simulink model "simple_AD_cont"  (R2019a)
settings: Solver=ode23tb  StartTime=0.0  StopTime=0.16  RelTol=1e-5  AbsTol=0.00001  EnableMultiTasking=on
values from neighbouring files (symbols this model uses):
  C_x1 = 10e-6    (= 1e-05)    [start.m]
  DEN_cc = Ks_curr.den{1,1}    [start.m]
  f_n = 50    [start.m]
  f_sw = 8000    [start.m]
  Id_ref = 15    [start.m]
  kic = ss(0,0,0,kic,Ts_control)    [current_controller.m]    (also in start.m = 0.042)
  L_f1 = 1.6e-3    (= 0.0016)    [start.m]
  L_f2 = 0.8e-3    (= 0.0008)    [start.m]
  Lgrid = 5e-3    (= 0.005)    [start.m]
  NUM_cc = Ks_curr.num{1,1}    [start.m]
  R_f1 = 2e-3    (= 0.002)    [start.m]
  R_f2 = 1e-3    (= 0.001)    [start.m]
  R_x1 = 0.1e-3    (= 0.0001)    [start.m]
  Rgrid = 10    [start.m]
  Ts_control = 1/f_sample    (= 6.25e-05)    [start.m]
  V_dc_ref = 700    [start.m]
  V_ffwd = -1    [start.m]
  Vg_h12 = 0*Vgrid    [start.m]
  Vg_h15 = 0*Vgrid    [start.m]
  Vg_h5 = 0*Vgrid    [start.m]
  Vg_h7 = 0*Vgrid    [start.m]
  Vgrid = 127*sqrt(2)    [start.m]
undefined symbols (not defined in the file or in its folder): C_f1, T_power
libraries: powerlib x21, simulink x2, powerlib_extras x2, powerlib_meascontrol x1
settings Model: Creator=FOR_WORK  LastModifiedBy=ityur
settings SolverCC: AutoScaleAbsTol=off
settings DataIOCC: LimitDataPoints=on  SaveFormat=Array  SignalLoggingSaveFormat=ModelDataLogs  ReturnWorkspaceOutputs=off
settings OptimizationCC: LifeSpan=inf
settings DebuggingCC: UnderspecifiedInitializationDetection=Classic  MergeDetectMultiDrivingBlocksExec=none  SolverPrmCheckMsg=warning  MultiTaskDSMMsg=warning  MultiTaskCondExecSysMsg=none  UnconnectedInputMsg=none  UnconnectedOutputMsg=none  UnconnectedLineMsg=none  StateNameClashWarn=warning  SFUnexpectedBacktrackingDiag=warning  SFNoUnconditionalDefaultTransitionDiag=warning  SFExecutionAtInitializationDiag=none  ArithmeticOperatorsInVariantConditions=warning
settings HardwareCC: ProdBitPerPointer=32  ProdBitPerSizeT=32  ProdBitPerPtrDiffT=32  ProdLargestAtomicFloat=None  ProdIntDivRoundTo=Undefined  ProdEndianess=Unspecified  ProdWordSize=32  ProdHWDeviceType=32-bit Generic
settings ModelReferenceCC: PropagateSignalLabelsOutOfModel=off
settings SFSimCC: SimUseLocalCustomCode=off
settings RTWCC: RTWUseLocalCustomCode=off
settings CodeAppCC: StateflowObjectComments=on
settings GRTTargetCC: TargetLangStandard=C89/C90 (ANSI)  GeneratePreprocessorConditionals=Disable all
settings ConfigComp: CovMetricSettings=dw  CovHtmlReporting=on  CovSaveCumulativeToWorkspaceVar=on  CovSaveSingleToWorkspaceVar=on  CovExternalEMLEnable=off  CovSFcnEnable=off
settings SimscapeCC: SimscapeNormalizeSystem=off

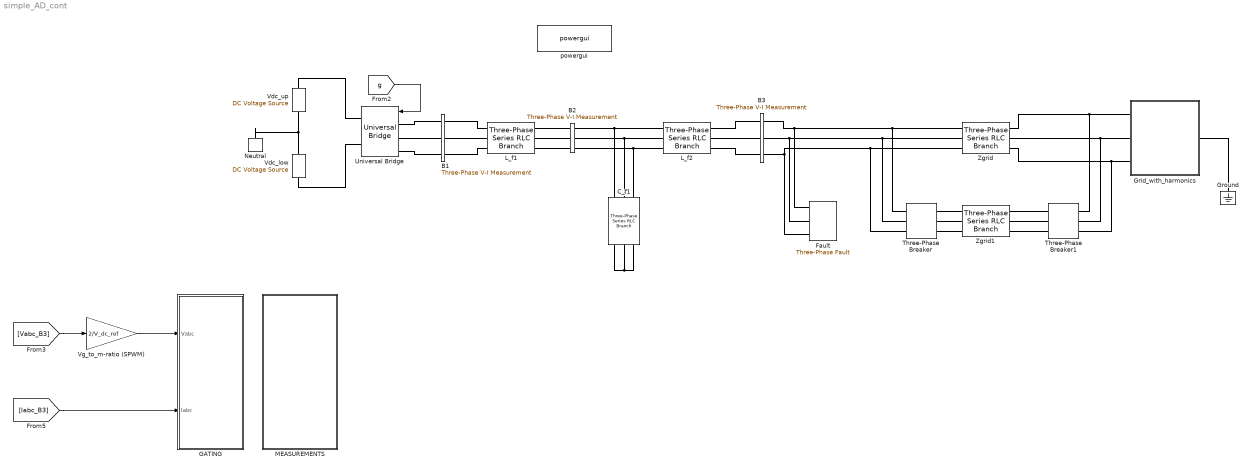
== system simple_AD_cont ==
  B1 : powerlib/Measurements/Three-Phase V-I Measurement  VoltageMeasurement=phase-to-phase  SetLabelV=on  LabelV=Vabc_B1  Vpu=off  VpuLL=off  CurrentMeasurement=yes  SetLabelI=on  LabelI=Iabc_B1  Ipu=off  Pbase=28e3  Vbase=480  OutputType=Magnitude  PhasorSimulation=off  PSBequivalent=0
      settings: SourceProductName=Simscape Electrical
  B2 : powerlib/Measurements/Three-Phase V-I Measurement  VoltageMeasurement=no  SetLabelV=on  LabelV=Vabc_B2  Vpu=off  VpuLL=off  CurrentMeasurement=yes  SetLabelI=on  LabelI=Iabc_B2  Ipu=off  Pbase=50e3  Vbase=Vi_n  OutputType=Magnitude  PhasorSimulation=off  PSBequivalent=0
      settings: SourceProductName=Simscape Electrical
  B3 : powerlib/Measurements/Three-Phase V-I Measurement  VoltageMeasurement=phase-to-ground  SetLabelV=on  LabelV=Vabc_B3  Vpu=off  VpuLL=off  CurrentMeasurement=yes  SetLabelI=on  LabelI=Iabc_B3  Ipu=off  Pbase=50e3  Vbase=Vi_n  OutputType=Magnitude  PhasorSimulation=off  PSBequivalent=0
      settings: SourceProductName=Simscape Electrical
  C_f1 : powerlib/Elements/Three-Phase Series RLC Branch  LConnTagsString=A|B|C  RConnTagsString=A|B|C  BranchType=RC  Resistance=R_x1  Inductance=L_f1  Capacitance=C_x1  Measurements=None
      settings: SourceProductName=Simscape Electrical
  Fault : powerlib/Elements/Three-Phase Fault  InitialStates=0  FaultA=on  FaultB=on  FaultC=on  GroundFault=on  SwitchTimes=[0.08 0.12]  External=off  SwitchStatus=NaN  FaultResistance=1e-9  GroundResistance=0.001  SnubberResistance=1e6  SnubberCapacitance=inf  Measurements=Fault voltages
      settings: SourceProductName=Simscape Electrical
  GATING : Subsystem
  Grid_with_harmonics : Subsystem
  Ground : powerlib/Elements/Ground  LConnTagsString=a
      settings: SourceProductName=Simscape Electrical
  L_f1 : powerlib/Elements/Three-Phase Series RLC Branch  LConnTagsString=A|B|C  RConnTagsString=A|B|C  BranchType=RL  Resistance=R_f1  Inductance=L_f1  Capacitance=C_f1  Measurements=None
      settings: SourceProductName=Simscape Electrical
  L_f2 : powerlib/Elements/Three-Phase Series RLC Branch  LConnTagsString=A|B|C  RConnTagsString=A|B|C  BranchType=RL  Resistance=R_f2  Inductance=L_f2  Capacitance=C_f1  Measurements=None
      settings: SourceProductName=Simscape Electrical
  MEASUREMENTS : Subsystem
  Neutral : powerlib/Elements/Neutral  LConnTagsString=a  NodeNumber=1
      settings: SourceProductName=Simscape Electrical  SourceProductBaseCode=PS
  Three-Phase Breaker : powerlib/Elements/Three-Phase Breaker  InitialState=open  SwitchA=on  SwitchB=on  SwitchC=on  SwitchTimes=111  External=off  BreakerResistance=0.0001  SnubberResistance=1e6  SnubberCapacitance=inf  Measurements=None
      settings: SourceProductName=Simscape Electrical
  Three-Phase Breaker1 : powerlib/Elements/Three-Phase Breaker  InitialState=open  SwitchA=on  SwitchB=on  SwitchC=on  SwitchTimes=111  External=off  BreakerResistance=0.0001  SnubberResistance=1e6  SnubberCapacitance=inf  Measurements=None
      settings: SourceProductName=Simscape Electrical
  Universal Bridge : powerlib/Power Electronics/Universal Bridge  Arms=3  SnubberResistance=1e5  SnubberCapacitance=inf  Device=Ideal Switches  Ron=1e-3  Lon=0  ForwardVoltages="[  0  0  ]"  ForwardVoltage=0  GTOparameters=[ 10e-6 , 20e-6 ]  IGBTparameters=[ 1e-6 , 2e-6 ]  Measurements=None  Measurements_2=None  converterType=Rectifier
      settings: SourceProductName=Simscape Electrical
  Vdc_low : powerlib/Electrical Sources/DC Voltage Source  Amplitude=V_dc_ref/2  Measurements=None
      settings: SourceProductName=Simscape Electrical
  Vdc_up : powerlib/Electrical Sources/DC Voltage Source  Amplitude=V_dc_ref/2  Measurements=None
      settings: SourceProductName=Simscape Electrical
  Vg_to_m-ratio (SPWM) : Gain  Gain=2/V_dc_ref
  Zgrid : powerlib/Elements/Three-Phase Series RLC Branch  LConnTagsString=A|B|C  RConnTagsString=A|B|C  BranchType=RL  Resistance=Rgrid  Inductance=Lgrid  Capacitance=C_f1  Measurements=None
      settings: SourceProductName=Simscape Electrical
  Zgrid1 : powerlib/Elements/Three-Phase Series RLC Branch  LConnTagsString=A|B|C  RConnTagsString=A|B|C  BranchType=R  Resistance=0.0001  Inductance=0  Capacitance=C_f1  Measurements=None
      settings: SourceProductName=Simscape Electrical
  powergui : powerlib/powergui  Priority=1  SimulationMode=Continuous  SampleTime=T_power  frequency=60  Iterations=50  frequencyindice=0  Pbase=100e6  ErrMax=1e-4  UnitsV=kV  UnitsW=MW  buscounter=0  FunctionMessages=off  echomessages=off  EnableUseOfTLC=off  CurrentSourceSwitches=on  DisableSnubberDevices=off  DisableRonSwitches=off  DisableVfSwitches=off  DisplayEquations=off  AutomaticDiscreteSolvers=off  SolverType=Tustin  Interpol=off  ExternalGateDelay=off  methode=off  Ts=0  x0status=blocks  SPID=off  SwTol=0  HookPort=off  NonlinearTolerance=0  nMaxIteration=15  ContinueOnMaxIteration=off  RestoreLinks=warning  ResistiveCurrentMeasurement=off  Frange=[0:2:500]  Ylog=off  Xlog=on  ShowGrid=off  save=off  variable=ZData  structure=Grid_Curr_THD  ZoomFFT=off  StartTime=0.2 - 2*0.02  cycles=2  DisplayStyle=1  fundamental=50  FreqAxis=off  MaxFrequency=1000  frequencyindicesteady=1  RmsSteady=1  display=off
      settings: SourceProductName=Simscape Electrical
  wires:
  [g] -> Universal Bridge/1
  [Iabc_B3] -> GATING/2(Iabc)
  [Vabc_B3] -> Vg_to_m-ratio (SPWM)/1
  Vg_to_m-ratio (SPWM)/1 -> GATING/1(Vabc)
  connections:
  Universal Bridge/LConn2 -- B1/LConn2
  B1/RConn2 -- L_f1/LConn2
  Universal Bridge/LConn1 -- B1/LConn1
  B1/RConn1 -- L_f1/LConn1
  Universal Bridge/LConn3 -- B1/LConn3
  B1/RConn3 -- L_f1/LConn3
  B3/RConn3 -- Three-Phase Breaker/LConn3 -- Zgrid/LConn3 -- Fault/LConn3
  B2/RConn1 -- C_f1/LConn1 -- L_f2/LConn1
  C_f1/RConn2 -- C_f1/RConn3 -- C_f1/RConn1
  L_f1/RConn2 -- B2/LConn2
  L_f1/RConn1 -- B2/LConn1
  L_f1/RConn3 -- B2/LConn3
  B3/RConn1 -- Three-Phase Breaker/LConn1 -- Zgrid/LConn1 -- Fault/LConn1
  B3/RConn2 -- Three-Phase Breaker/LConn2 -- Zgrid/LConn2 -- Fault/LConn2
  L_f2/RConn2 -- B3/LConn2
  L_f2/RConn1 -- B3/LConn1
  L_f2/RConn3 -- B3/LConn3
  Universal Bridge/RConn1 -- Vdc_up/RConn1
  Zgrid/RConn1 -- Three-Phase Breaker1/RConn1 -- Grid_with_harmonics/LConn1
  Zgrid/RConn2 -- Three-Phase Breaker1/RConn2 -- Grid_with_harmonics/LConn2
  Zgrid/RConn3 -- Three-Phase Breaker1/RConn3 -- Grid_with_harmonics/LConn3
  B2/RConn2 -- C_f1/LConn2 -- L_f2/LConn2
  B2/RConn3 -- C_f1/LConn3 -- L_f2/LConn3
  Vdc_up/LConn1 -- Neutral/LConn1 -- Vdc_low/RConn1
  Vdc_low/LConn1 -- Universal Bridge/RConn2
  Grid_with_harmonics/RConn1 -- Ground/LConn1
  Three-Phase Breaker/RConn1 -- Zgrid1/LConn1
  Three-Phase Breaker/RConn2 -- Zgrid1/LConn2
  Three-Phase Breaker/RConn3 -- Zgrid1/LConn3
  Zgrid1/RConn1 -- Three-Phase Breaker1/LConn1
  Zgrid1/RConn2 -- Three-Phase Breaker1/LConn2
  Zgrid1/RConn3 -- Three-Phase Breaker1/LConn3

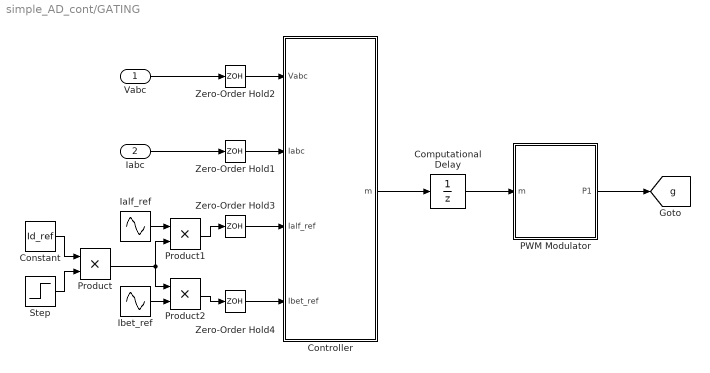
== system simple_AD_cont/GATING ==
  Vabc : Inport  PortDimensions=3
  Iabc : Inport  Port=2  PortDimensions=3
  Computational Delay : UnitDelay  SampleTime=Ts_control  HasFrameUpgradeWarning=on
  Constant : Constant  Value=Id_ref
  Controller : Subsystem
  Ialf_ref : Sin  Frequency=2*pi*f_n  SampleTime=0
  Ibet_ref : Sin  Frequency=2*pi*f_n  Phase=-pi/2  SampleTime=0
  PWM Modulator : Subsystem
  Product : Product
  Product1 : Product
  Product2 : Product
  Step : Step  Time=0.04  SampleTime=0
  Zero-Order Hold{1..4} (4 alike) : ZeroOrderHold  SampleTime=Ts_control
  tag scope: g=global
  wires:
  Zero-Order Hold2/1 -> Controller/1(Vabc)
  Vabc/1 -> Zero-Order Hold2/1
  PWM Modulator/1(P1) -> [g]
  Iabc/1 -> Zero-Order Hold1/1
  Controller/1(m) -> Computational Delay/1
  Computational Delay/1 -> PWM Modulator/1(m)
  Zero-Order Hold1/1 -> Controller/2(Iabc)
  Zero-Order Hold3/1 -> Controller/3(Ialf_ref)
  Zero-Order Hold4/1 -> Controller/4(Ibet_ref)
  Step/1 -> Product/2
  Constant/1 -> Product/1
  Ialf_ref/1 -> Product1/1
  Product1/1 -> Zero-Order Hold3/1
  Product2/1 -> Zero-Order Hold4/1
  Ibet_ref/1 -> Product2/2
  Product/1 -> Product2/1, Product1/2

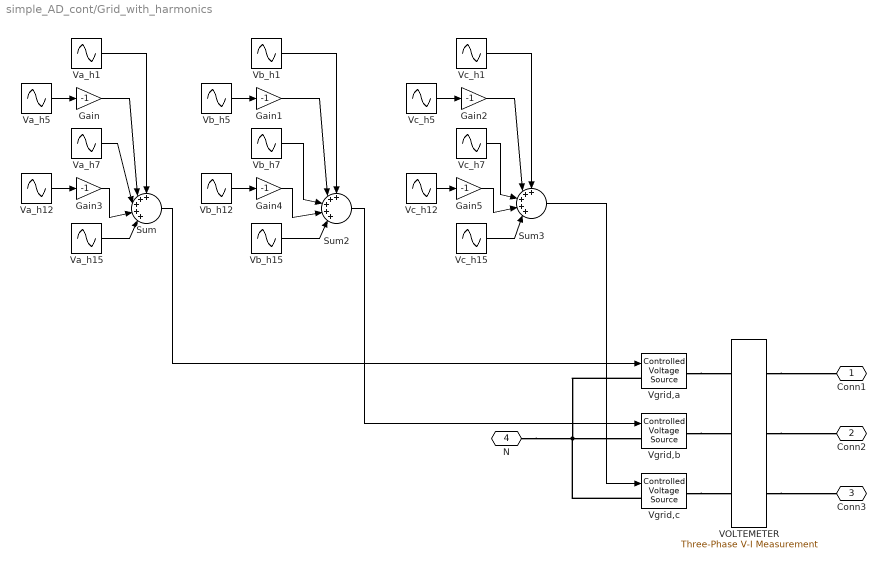
== system simple_AD_cont/Grid_with_harmonics ==
  Gain{,1..5} (6 alike) : Gain  Gain=-1
  Sum : Sum  Inputs=+++++|
  Sum2 : Sum  Inputs=+++++|
  Sum3 : Sum  Inputs=+++++|
  VOLTEMETER : powerlib/Measurements/Three-Phase V-I Measurement  VoltageMeasurement=phase-to-ground  SetLabelV=on  LabelV=V_grid  Vpu=off  VpuLL=off  CurrentMeasurement=no  SetLabelI=off  LabelI=Iabc  Ipu=off  Pbase=100e6  Vbase=500e3  OutputType=Complex  PhasorSimulation=off  PSBequivalent=0
      settings: SourceProductName=Simscape Electrical
  Va_h1 : Sin  Amplitude=Vgrid  Frequency=2*pi*f_n  SampleTime=0
  Va_h12 : Sin  Amplitude=Vg_h12  Frequency=12*2*pi*f_n  SampleTime=0
  Va_h15 : Sin  Amplitude=Vg_h15  Frequency=15*2*pi*f_n  SampleTime=0
  Va_h5 : Sin  Amplitude=Vg_h5  Frequency=5*2*pi*f_n  SampleTime=0
  Va_h7 : Sin  Amplitude=Vg_h7  Frequency=7*2*pi*f_n  SampleTime=0
  Vb_h1 : Sin  Amplitude=Vgrid  Frequency=2*pi*f_n  Phase=-2*pi/3  SampleTime=0
  Vb_h12 : Sin  Amplitude=Vg_h12  Frequency=12*2*pi*f_n  Phase=2*pi/3  SampleTime=0
  Vb_h15 : Sin  Amplitude=Vg_h15  Frequency=15*2*pi*f_n  Phase=-2*pi/3  SampleTime=0
  Vb_h5 : Sin  Amplitude=Vg_h5  Frequency=5*2*pi*f_n  Phase=2*pi/3  SampleTime=0
  Vb_h7 : Sin  Amplitude=Vg_h7  Frequency=7*2*pi*f_n  Phase=-2*pi/3  SampleTime=0
  Vc_h1 : Sin  Amplitude=Vgrid  Frequency=2*pi*f_n  Phase=2*pi/3  SampleTime=0
  Vc_h12 : Sin  Amplitude=Vg_h12  Frequency=12*2*pi*f_n  Phase=-2*pi/3  SampleTime=0
  Vc_h15 : Sin  Amplitude=Vg_h15  Frequency=15*2*pi*f_n  Phase=2*pi/3  SampleTime=0
  Vc_h5 : Sin  Amplitude=Vg_h5  Frequency=5*2*pi*f_n  Phase=-2*pi/3  SampleTime=0
  Vc_h7 : Sin  Amplitude=Vg_h7  Frequency=7*2*pi*f_n  Phase=2*pi/3  SampleTime=0
  Vgrid,a : powerlib/Electrical Sources/Controlled Voltage Source  Initialize=on  Source_Type=AC  Amplitude=0  Phase=0  Frequency=0  Measurements=None
      settings: SourceProductName=Simscape Electrical
  Vgrid,b : powerlib/Electrical Sources/Controlled Voltage Source  Initialize=on  Source_Type=AC  Amplitude=0  Phase=0  Frequency=0  Measurements=None
      settings: SourceProductName=Simscape Electrical
  Vgrid,c : powerlib/Electrical Sources/Controlled Voltage Source  Initialize=on  Source_Type=AC  Amplitude=0  Phase=0  Frequency=0  Measurements=None
      settings: SourceProductName=Simscape Electrical
  Conn1 : PMIOPort  Side=Left
  Conn2 : PMIOPort  Port=2  Side=Left
  Conn3 : PMIOPort  Port=3  Side=Left
  N : PMIOPort  Port=4  Side=Right
  wires:
  Va_h1/1 -> Sum/1
  Va_h5/1 -> Gain/1
  Va_h7/1 -> Sum/3
  Va_h12/1 -> Gain3/1
  Va_h15/1 -> Sum/5
  Vb_h1/1 -> Sum2/1
  Vb_h5/1 -> Gain1/1
  Vb_h7/1 -> Sum2/3
  Vb_h12/1 -> Gain4/1
  Vb_h15/1 -> Sum2/5
  Vc_h1/1 -> Sum3/1
  Vc_h5/1 -> Gain2/1
  Vc_h7/1 -> Sum3/3
  Vc_h12/1 -> Gain5/1
  Vc_h15/1 -> Sum3/5
  Sum/1 -> Vgrid,a/1
  Sum2/1 -> Vgrid,b/1
  Sum3/1 -> Vgrid,c/1
  Gain/1 -> Sum/2
  Gain1/1 -> Sum2/2
  Gain2/1 -> Sum3/2
  Gain3/1 -> Sum/4
  Gain4/1 -> Sum2/4
  Gain5/1 -> Sum3/4
  connections:
  Vgrid,a/LConn1 -- N/RConn1 -- Vgrid,c/LConn1 -- Vgrid,b/LConn1
  Vgrid,a/RConn1 -- VOLTEMETER/LConn1
  Vgrid,b/RConn1 -- VOLTEMETER/LConn2
  Vgrid,c/RConn1 -- VOLTEMETER/LConn3
  VOLTEMETER/RConn3 -- Conn3/RConn1
  VOLTEMETER/RConn2 -- Conn2/RConn1
  VOLTEMETER/RConn1 -- Conn1/RConn1

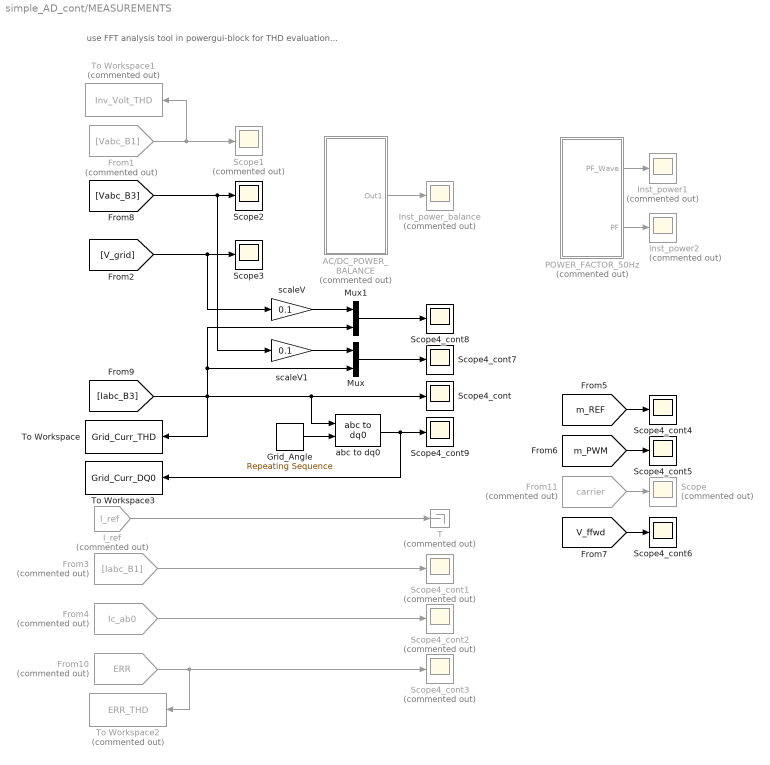
== system simple_AD_cont/MEASUREMENTS ==
  note: use FFT analysis tool in powergui-block
      |  for THD evaluation...
  AC/DC_POWER_BALANCE : Subsystem  Commented=on
  From1 : From  Commented=on  GotoTag=Vabc_B1  TagVisibility=global
      settings: CloseFcn=tagdialog Close
  From10 : From  Commented=on  GotoTag=ERR  TagVisibility=global
      settings: CloseFcn=tagdialog Close
  From11 : From  Commented=on  GotoTag=carrier  TagVisibility=global
      settings: CloseFcn=tagdialog Close
  From3 : From  Commented=on  GotoTag=Iabc_B1  TagVisibility=global
      settings: CloseFcn=tagdialog Close
  From4 : From  Commented=on  GotoTag=Ic_ab0  TagVisibility=global
      settings: CloseFcn=tagdialog Close
  Grid_Angle : simulink/Sources/Repeating Sequence  rep_seq_t=[0 0.02]  rep_seq_y=[0 2*pi]
  I_ref : From  Commented=on  GotoTag=I_ref  TagVisibility=global
  Inst_power1 : Scope  Commented=on
  Inst_power2 : Scope  Commented=on
  Inst_power_balance : Scope  Commented=on
  Mux : Mux  Inputs=2
  Mux1 : Mux  Inputs=2
  POWER_FACTOR_50Hz : Subsystem  Commented=on
  Scope : Scope  Commented=on
  Scope1 : Scope  Commented=on
  Scope2 : Scope
  Scope3 : Scope
  Scope4_cont{,4..9} (7 alike) : Scope
  Scope4_cont1 : Scope  Commented=on
  Scope4_cont2 : Scope  Commented=on
  Scope4_cont3 : Scope  Commented=on
  T : Terminator  Commented=on
  To Workspace : ToWorkspace  VariableName=Grid_Curr_THD  SaveFormat=Structure With Time  SampleTime=-1
  To Workspace1 : ToWorkspace  Commented=on  VariableName=Inv_Volt_THD  SaveFormat=Structure With Time  SampleTime=-1
  To Workspace2 : ToWorkspace  Commented=on  VariableName=ERR_THD  SaveFormat=Structure With Time  SampleTime=-1
  To Workspace3 : ToWorkspace  VariableName=Grid_Curr_DQ0  SaveFormat=Structure With Time  SampleTime=-1
  abc to dq0 : powerlib_meascontrol/Transformations/abc to dq0  Alignment=90 degrees behind phase A axis
      settings: SourceProductName=Simscape Electrical
  scaleV : Gain  Gain=0.1
  scaleV1 : Gain  Gain=0.1
  wires:
  [V_grid] -> Scope3/1, scaleV/1
  [Iabc_B3] -> abc to dq0/1, Scope4_cont/1, To Workspace/1, Mux/2, Mux1/2
  From1/1 -> To Workspace1/1, Scope1/1
  [Vabc_B3] -> scaleV1/1, Scope2/1
  AC/DC_POWER_BALANCE/1(Out1) -> Inst_power_balance/1
  POWER_FACTOR_50Hz/1(PF_Wave) -> Inst_power1/1
  POWER_FACTOR_50Hz/2(PF) -> Inst_power2/1
  From3/1 -> Scope4_cont1/1
  From4/1 -> Scope4_cont2/1
  From10/1 -> To Workspace2/1, Scope4_cont3/1
  [V_ffwd] -> Scope4_cont6/1
  [m_PWM] -> Scope4_cont5/1
  [m_REF] -> Scope4_cont4/1
  I_ref/1 -> T/1
  Mux/1 -> Scope4_cont7/1
  Mux1/1 -> Scope4_cont8/1
  From11/1 -> Scope/1
  scaleV/1 -> Mux1/1
  scaleV1/1 -> Mux/1
  abc to dq0/1 -> To Workspace3/1, Scope4_cont9/1
  Grid_Angle/1 -> abc to dq0/2

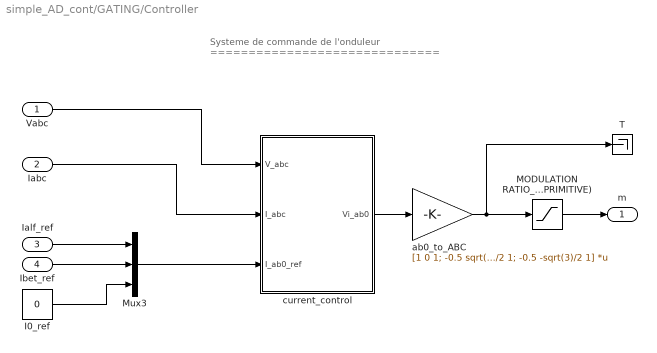
== system simple_AD_cont/GATING/Controller ==
  note: Systeme de commande de l'onduleur
      | ==============================
  Vabc : Inport  PortDimensions=3
  Iabc : Inport  Port=2  PortDimensions=3
  Ialf_ref : Inport  Port=3  PortDimensions=1
  Ibet_ref : Inport  Port=4  PortDimensions=1
  I0_ref : Constant  Value=0  SampleTime=Ts_control
  MODULATION RATIO_LIMITER (PRIMITIVE) : Saturate  UpperLimit=1  LowerLimit=-1
  Mux3 : Mux  Inputs=3
  T : Terminator
  ab0_to_ABC : Gain  Gain=[1 0 1; -0.5 sqrt(3)/2 1; -0.5 -sqrt(3)/2 1]  Multiplication=Matrix(K*u)
  current_control : Subsystem
  m : Outport
  wires:
  Vabc/1 -> current_control/1(V_abc)
  Mux3/1 -> current_control/3(I_ab0_ref)
  Iabc/1 -> current_control/2(I_abc)
  Ibet_ref/1 -> Mux3/2
  I0_ref/1 -> Mux3/3
  Ialf_ref/1 -> Mux3/1
  current_control/1(Vi_ab0) -> ab0_to_ABC/1
  ab0_to_ABC/1 -> T/1, MODULATION RATIO_LIMITER (PRIMITIVE)/1
  MODULATION RATIO_LIMITER (PRIMITIVE)/1 -> m/1

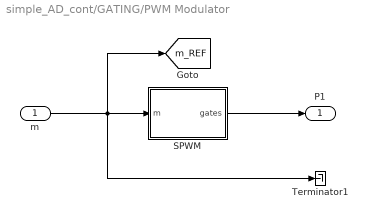
== system simple_AD_cont/GATING/PWM Modulator ==
  m : Inport
  SPWM : Subsystem
  Terminator1 : Terminator
  P1 : Outport
  tag scope: m_REF=global
  wires:
  m/1 -> [m_REF], SPWM/1(m), Terminator1/1
  SPWM/1(gates) -> P1/1

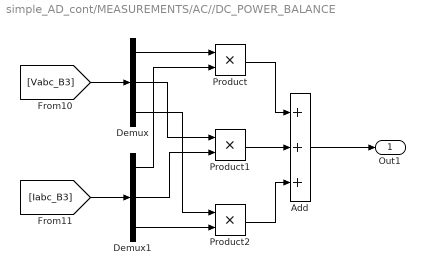
== system simple_AD_cont/MEASUREMENTS/AC//DC_POWER_BALANCE ==
  Add : Sum  Inputs=+++
  Demux : Demux  Outputs=3
  Demux1 : Demux  Outputs=3
  Product : Product
  Product1 : Product
  Product2 : Product
  Out1 : Outport
  wires:
  Demux/1 -> Product/1
  Demux1/1 -> Product/2
  Demux/2 -> Product1/1
  Demux1/2 -> Product1/2
  Demux1/3 -> Product2/2
  Demux/3 -> Product2/1
  Product1/1 -> Add/2
  Product/1 -> Add/1
  Product2/1 -> Add/3
  Add/1 -> Out1/1
  [Iabc_B3] -> Demux1/1
  [Vabc_B3] -> Demux/1

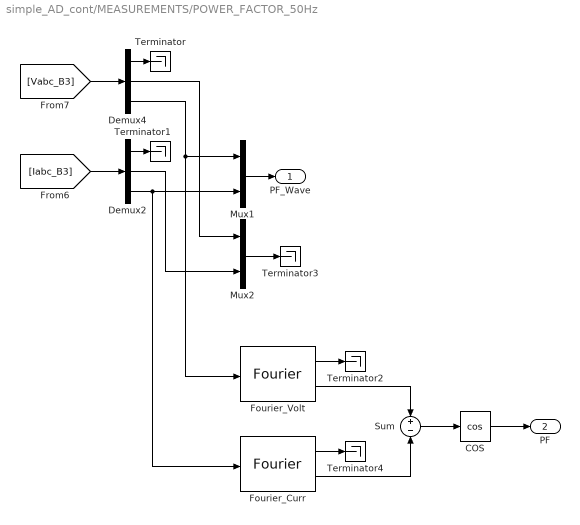
== system simple_AD_cont/MEASUREMENTS/POWER_FACTOR_50Hz ==
  COS : Trigonometry  Operator=cos
  Demux2 : Demux  Outputs=3
  Demux4 : Demux  Outputs=3
  Fourier_Curr : powerlib_extras/Measurements/Fourier  f1=50  n=1
      settings: SourceProductName=Simscape Electrical  SourceProductBaseCode=PS
  Fourier_Volt : powerlib_extras/Measurements/Fourier  f1=50  n=1
      settings: SourceProductName=Simscape Electrical  SourceProductBaseCode=PS
  Mux1 : Mux  Inputs=2
  Mux2 : Mux  Inputs=2
  Sum : Sum  Inputs=+|-
  Terminator{,1..4} (5 alike) : Terminator
  PF_Wave : Outport
  PF : Outport  Port=2
  wires:
  Mux1/1 -> PF_Wave/1
  Demux4/3 -> Mux1/1, Fourier_Volt/1
  Demux4/2 -> Mux2/1
  Demux4/1 -> Terminator/1
  [Iabc_B3] -> Demux2/1
  Demux2/1 -> Terminator1/1
  [Vabc_B3] -> Demux4/1
  Mux2/1 -> Terminator3/1
  Demux2/3 -> Fourier_Curr/1, Mux1/2
  Demux2/2 -> Mux2/2
  Fourier_Volt/1 -> Terminator2/1
  Fourier_Curr/1 -> Terminator4/1
  Fourier_Volt/2 -> Sum/1
  Fourier_Curr/2 -> Sum/2
  Sum/1 -> COS/1
  COS/1 -> PF/1

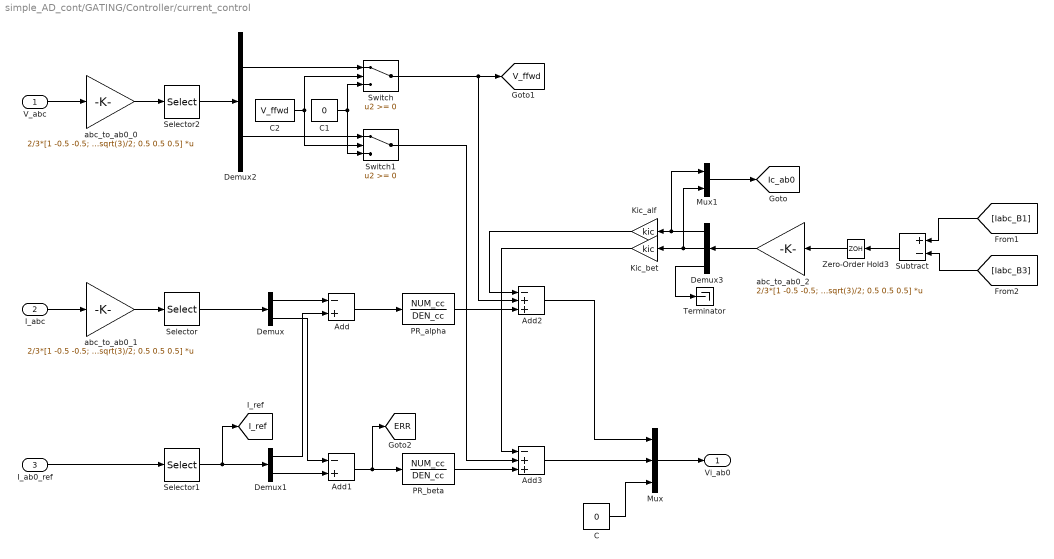
== system simple_AD_cont/GATING/Controller/current_control ==
  V_abc : Inport
  I_abc : Inport  Port=2
  I_ab0_ref : Inport  Port=3
  Add : Sum  Inputs=-+
  Add1 : Sum  Inputs=-+
  Add2 : Sum  Inputs=-++
  Add3 : Sum  Inputs=-++
  C : Constant  Value=0  SampleTime=Ts_control
  C1 : Constant  Value=0  SampleTime=Ts_control
  C2 : Constant  Value=V_ffwd  SampleTime=Ts_control
  Demux : Demux  Outputs=2
  Demux1 : Demux  Outputs=2
  Demux2 : Demux  Outputs=2
  Demux3 : Demux  Outputs=3
  Kic_alf : Gain  Gain=kic
  Kic_bet : Gain  Gain=kic
  Mux : Mux  Inputs=3
  Mux1 : Mux  Inputs=2
  PR_alpha : DiscreteTransferFcn  Numerator=NUM_cc  Denominator=DEN_cc  SampleTime=Ts_control
  PR_beta : DiscreteTransferFcn  Numerator=NUM_cc  Denominator=DEN_cc  SampleTime=Ts_control
  Selector : Selector  InputPortWidth=3  IndexOptions=Index vector (dialog)  Indices=[1 2]  OutputSizes=1
  Selector1 : Selector  InputPortWidth=3  IndexOptions=Index vector (dialog)  Indices=[1 2]  OutputSizes=1
  Selector2 : Selector  InputPortWidth=3  IndexOptions=Index vector (dialog)  Indices=[1 2]  OutputSizes=1
  Subtract : Sum  Inputs=+-
  Switch : Switch
  Switch1 : Switch
  Terminator : Terminator
  Zero-Order Hold3 : ZeroOrderHold  SampleTime=Ts_control
  abc_to_ab0_0 : Gain  Gain=2/3*[1 -0.5 -0.5; 0 sqrt(3)/2 -sqrt(3)/2; 0.5 0.5 0.5]  Multiplication=Matrix(K*u)
  abc_to_ab0_1 : Gain  Gain=2/3*[1 -0.5 -0.5; 0 sqrt(3)/2 -sqrt(3)/2; 0.5 0.5 0.5]  Multiplication=Matrix(K*u)
  abc_to_ab0_2 : Gain  Gain=2/3*[1 -0.5 -0.5; 0 sqrt(3)/2 -sqrt(3)/2; 0.5 0.5 0.5]  Multiplication=Matrix(K*u)
  Vi_ab0 : Outport
  tag scope: ERR=global, I_ref=global, Ic_ab0=global, V_ffwd=global
  wires:
  I_abc/1 -> abc_to_ab0_1/1
  abc_to_ab0_1/1 -> Selector/1
  Selector/1 -> Demux/1
  Selector1/1 -> [I_ref], Demux1/1
  Demux1/1 -> Add/2
  Demux/1 -> Add/1
  Demux1/2 -> Add1/2
  Demux/2 -> Add1/1
  Add/1 -> PR_alpha/1
  C/1 -> Mux/3
  Mux/1 -> Vi_ab0/1
  Add1/1 -> [ERR], PR_beta/1
  V_abc/1 -> abc_to_ab0_0/1
  abc_to_ab0_0/1 -> Selector2/1
  Selector2/1 -> Demux2/1
  Switch/1 -> [V_ffwd], Add2/2
  Add3/1 -> Mux/2
  Add2/1 -> Mux/1
  C1/1 -> Switch/3, Switch1/3
  C2/1 -> Switch1/2, Switch/2
  Demux2/1 -> Switch/1
  Demux2/2 -> Switch1/1
  I_ab0_ref/1 -> Selector1/1
  PR_alpha/1 -> Add2/3
  abc_to_ab0_2/1 -> Demux3/1
  Demux3/1 -> Mux1/1, Kic_alf/1
  PR_beta/1 -> Add3/3
  Switch1/1 -> Add3/2
  Demux3/2 -> Mux1/2, Kic_bet/1
  Demux3/3 -> Terminator/1
  Kic_alf/1 -> Add2/1
  Kic_bet/1 -> Add3/1
  Mux1/1 -> [Ic_ab0]
  [Iabc_B3] -> Subtract/2
  Subtract/1 -> Zero-Order Hold3/1
  Zero-Order Hold3/1 -> abc_to_ab0_2/1
  [Iabc_B1] -> Subtract/1

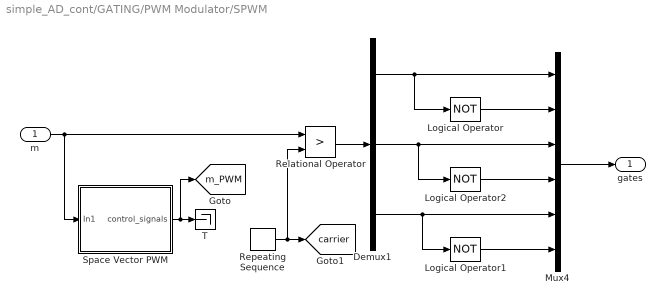
== system simple_AD_cont/GATING/PWM Modulator/SPWM ==
  m : Inport
  Demux1 : Demux  Outputs=3
  Logical Operator : Logic  Operator=NOT  AllPortsSameDT=off  OutDataTypeStr=boolean
  Logical Operator1 : Logic  Operator=NOT  AllPortsSameDT=off  OutDataTypeStr=boolean
  Logical Operator2 : Logic  Operator=NOT  AllPortsSameDT=off  OutDataTypeStr=boolean
  Mux4 : Mux  Inputs=6
  Relational Operator : RelationalOperator  Operator=>  RndMeth=Nearest
  Repeating Sequence : simulink/Sources/Repeating Sequence  rep_seq_t=[0 0.25/f_sw 0.5/f_sw 0.75/f_sw 1/f_sw]  rep_seq_y=[-1 0 1 0 -1]
  Space Vector PWM : Subsystem
  T : Terminator
  gates : Outport
  tag scope: carrier=global, m_PWM=global
  wires:
  Repeating Sequence/1 -> [carrier], Relational Operator/2
  Demux1/1 -> Logical Operator/1, Mux4/1
  Logical Operator/1 -> Mux4/2
  m/1 -> Space Vector PWM/1(In1), Relational Operator/1
  Demux1/3 -> Logical Operator1/1, Mux4/5
  Relational Operator/1 -> Demux1/1
  Mux4/1 -> gates/1
  Logical Operator1/1 -> Mux4/6
  Demux1/2 -> Logical Operator2/1, Mux4/3
  Logical Operator2/1 -> Mux4/4
  Space Vector PWM/1(control_signals) -> [m_PWM], T/1

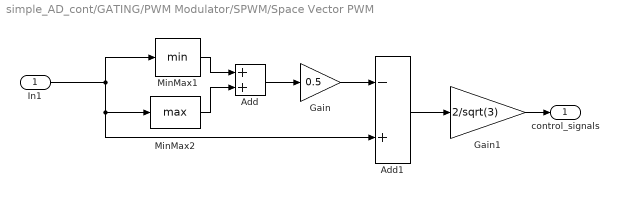
== system simple_AD_cont/GATING/PWM Modulator/SPWM/Space Vector PWM ==
  In1 : Inport
  Add : Sum
  Add1 : Sum  Inputs=-+
  Gain : Gain  Gain=0.5
  Gain1 : Gain  Gain=2/sqrt(3)
  MinMax1 : MinMax  SaturateOnIntegerOverflow=on  InputSameDT=on
  MinMax2 : MinMax  Function=max  SaturateOnIntegerOverflow=on  InputSameDT=on
  control_signals : Outport
  wires:
  In1/1 -> MinMax1/1, MinMax2/1, Add1/2
  MinMax1/1 -> Add/1
  MinMax2/1 -> Add/2
  Add/1 -> Gain/1
  Gain/1 -> Add1/1
  Add1/1 -> Gain1/1
  Gain1/1 -> control_signals/1
